simulink model "speed_torque_theta_v1_1"  (R2021a)
settings: Solver=VariableStepAuto  StartTime=0.0  StopTime=10.0  RelTol=1e-3
settings Model: Creator=danesh  LastModifiedBy=danesh

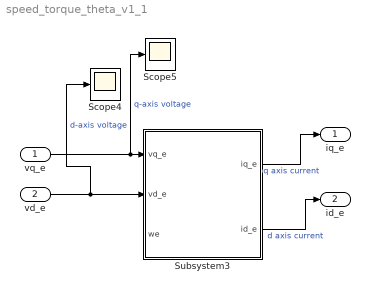
== system speed_torque_theta_v1_1 ==
  vq_e : Inport
  vd_e : Inport  Port=2
  Scope4 : Scope
  Scope5 : Scope
  Subsystem3 : Subsystem
  iq_e : Outport  VectorParamsAs1DForOutWhenUnconnected=off
  id_e : Outport  Port=2  VectorParamsAs1DForOutWhenUnconnected=off
  wires:
  Subsystem3/2(id_e) -> id_e/1  "d axis current"
  vq_e/1 -> Scope5/1, Subsystem3/1(vq_e)  "q-axis voltage"
  Subsystem3/1(iq_e) -> iq_e/1  "q axis current"
  vd_e/1 -> Scope4/1, Subsystem3/2(vd_e)  "d-axis voltage"

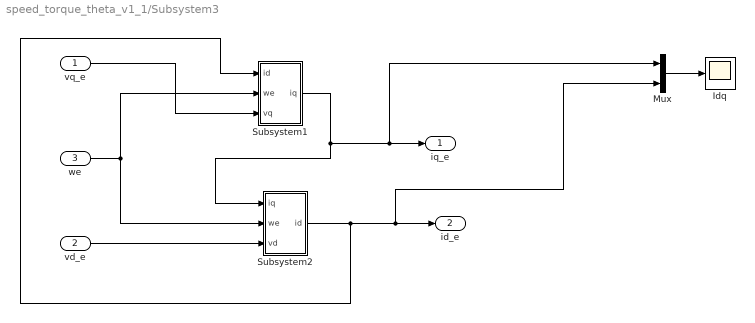
== system speed_torque_theta_v1_1/Subsystem3 ==
  vq_e : Inport
  vd_e : Inport  Port=2
  we : Inport  Port=3
  Idq : Scope
  Mux : Mux  Inputs=2
  Subsystem1 : Subsystem
  Subsystem2 : Subsystem
  iq_e : Outport  VectorParamsAs1DForOutWhenUnconnected=off
  id_e : Outport  Port=2  VectorParamsAs1DForOutWhenUnconnected=off
  wires:
  vq_e/1 -> Subsystem1/3(vq)
  vd_e/1 -> Subsystem2/3(vd)
  we/1 -> Subsystem1/2(we), Subsystem2/2(we)
  Subsystem1/1(iq) -> Subsystem2/1(iq), Mux/1, iq_e/1
  Subsystem2/1(id) -> Subsystem1/1(id), Mux/2, id_e/1
  Mux/1 -> Idq/1

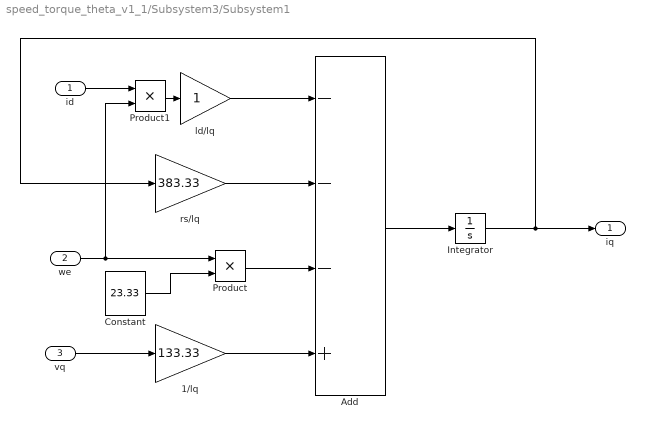
== system speed_torque_theta_v1_1/Subsystem3/Subsystem1 ==
  id : Inport
  we : Inport  Port=2
  vq : Inport  Port=3
  "1/lq " : Gain  Gain=133.33
  Add : Sum  Inputs=---+
  Constant : Constant  Value=23.33
  Integrator : Integrator
  Product : Product  RndMeth=Zero
  Product1 : Product  RndMeth=Zero
  "ld/lq " : Gain
  rs/lq : Gain  Gain=383.33
  iq : Outport  VectorParamsAs1DForOutWhenUnconnected=off
  wires:
  vq/1 -> "1/lq "/1
  "ld/lq "/1 -> Add/1
  rs/lq/1 -> Add/2
  "1/lq "/1 -> Add/4
  Add/1 -> Integrator/1
  Integrator/1 -> rs/lq/1, iq/1
  Product/1 -> Add/3
  we/1 -> Product/1, Product1/2
  Constant/1 -> Product/2
  Product1/1 -> "ld/lq "/1
  id/1 -> Product1/1

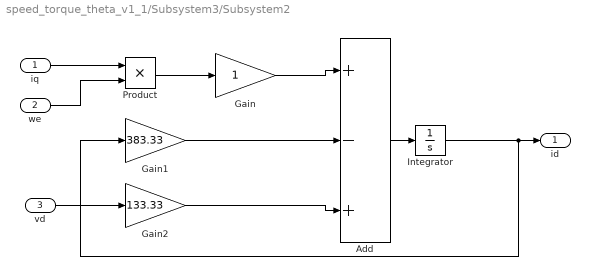
== system speed_torque_theta_v1_1/Subsystem3/Subsystem2 ==
  iq : Inport
  we : Inport  Port=2
  vd : Inport  Port=3
  Add : Sum  Inputs=+-+
  Gain : Gain
  Gain1 : Gain  Gain=383.33
  Gain2 : Gain  Gain=133.33
  Integrator : Integrator
  Product : Product  RndMeth=Zero
  id : Outport  VectorParamsAs1DForOutWhenUnconnected=off
  wires:
  iq/1 -> Product/1
  we/1 -> Product/2
  Product/1 -> Gain/1
  Gain/1 -> Add/1
  Add/1 -> Integrator/1
  Gain1/1 -> Add/2
  vd/1 -> Gain2/1
  Gain2/1 -> Add/3
  Integrator/1 -> Gain1/1, id/1
